simulink library "fcnLib4joint_sim"  (R2018b)
settings: Solver=VariableStepAuto  StartTime=0.0  StopTime=10.0  RelTol=1e-3
values from neighbouring files (symbols this model uses):
  alpha = 1.0    (= 1)    [init.m]
  D_el = 0    [init.m]
  F_c = 35    [init.m]
  F_s = 40    [init.m]
  J_joint = 4.155    [init.m]
  J_load = 1.2252    [init.m]
  K0_colli = 100    [init.m]
  K_el = 6900    [init.m]
  L_fricObs = 50    [init.m]
  sigma0 = 2000    [init.m]
  sigma1 = 200    [init.m]
  sigma2 = D_visc    (= 20)    [init.m]
  vs = 0.1    [init.m]
undefined symbols (not defined in the file or in its folder): threshold_colli, X, Y, Z
libraries: fl_lib x22, nesl_utility x16, sm_lib x6, simulink x4, sdl_lib x2, dsparch4 x1
settings Model: Creator=qiming  LastModifiedBy=qiming

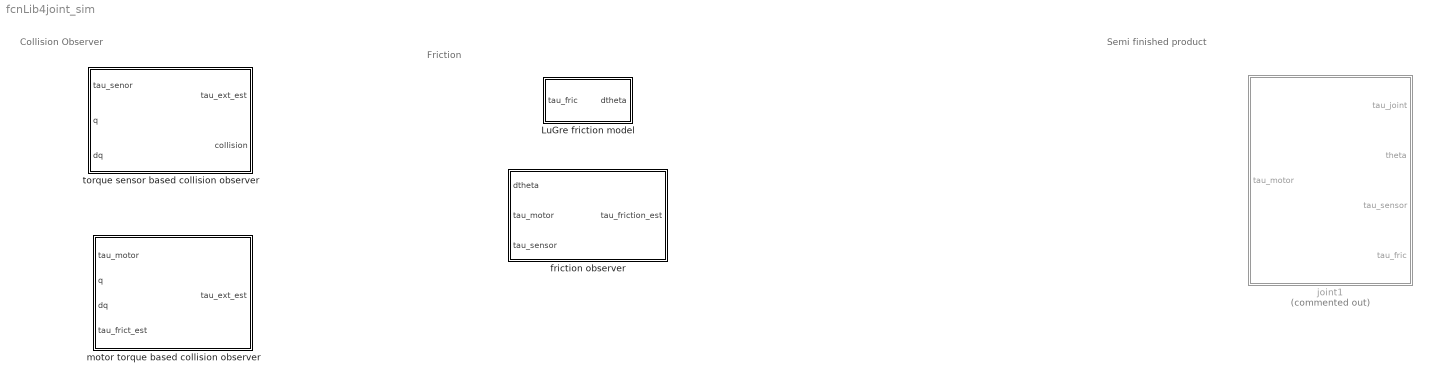
== system fcnLib4joint_sim ==
  note: Semi finished product
  note: Friction
  note: Collision Observer
  " torque sensor based collision observer " : Subsystem
  LuGre friction model : Subsystem
  friction observer : Subsystem
  joint1 : Subsystem  Commented=on
  motor torque based collision observer : Subsystem

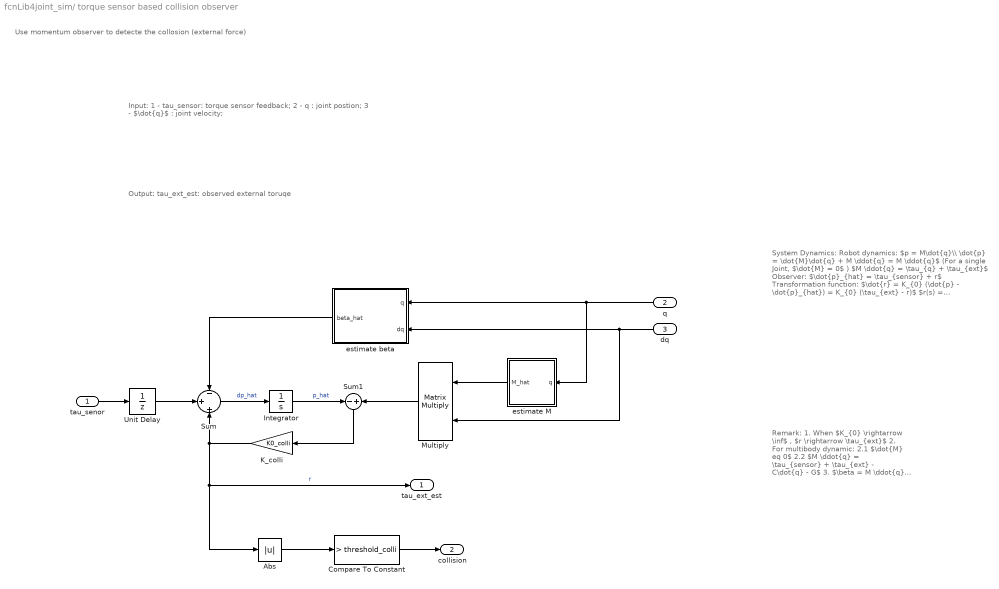
== system fcnLib4joint_sim/ torque sensor based collision observer  ==
  note: Input:
      | 1 - tau_sensor: torque sensor feedback;
      | 2 - q : joint postion;
      | 3 - $\dot{q}$ : joint velocity;
  note: Use momentum observer to detecte the collosion (external force)
  note: Output:
      | tau_ext_est: observed external toruqe
  note: System Dynamics:
      | Robot dynamics:
      | $p = M\dot{q}\\ \dot{p} = \dot{M}\dot{q} + M \ddot{q} = M \ddot{q}$ (For a single Joint, $\dot{M} = 0$ )
      | $M \ddot{q} = \tau_{q} + \tau_{ext}$
      | Observer:
      | $\dot{p}_{hat} = \tau_{sensor} + r$
      | Transformation function:
      | $\dot{r} = K_{0} (\dot{p} - \dot{p}_{hat}) = K_{0} (\tau_{ext} - r)$
      | $r(s) = \frac{1}{1+\frac{1}{K_{0}}s} \tau_{ext}(s)$
  note: Remark:
      | 1. When $K_{0} \rightarrow \inf$ , $r \rightarrow \tau_{ext}$
      | 2. For multibody dynamic:
      | 2.1 $\dot{M} \neq 0$
      | 2.2 $M \ddot{q} = \tau_{sensor} + \tau_{ext} - C\dot{q} - G$
      | 3. $\beta = M \ddot{q} = C\dot{q} + G$
  tau_senor : Inport
  q : Inport  Port=2
  dq : Inport  Port=3
  Abs : Abs
  Compare To Constant : simulink/Logic and Bit Operations/Compare To Constant  relop=>  const=threshold_colli  OutDataTypeStr=boolean
  Integrator : Integrator
  K_colli : Gain  Gain=K0_colli
  Multiply : Product  Multiplication=Matrix(*)
  Sum : Sum  Inputs=-|+|+
  Sum1 : Sum  Inputs=-+
  Unit Delay : UnitDelay  SampleTime=-1
  estimate M : Subsystem
  "estimate beta " : Subsystem
  tau_ext_est : Outport
  collision : Outport  Port=2
  wires:
  tau_senor/1 -> Unit Delay/1
  q/1 -> estimate M/1(q), "estimate beta "/1(q)
  "estimate beta "/1(beta_hat) -> Sum/1
  Sum/1 -> Integrator/1  "dp_hat"
  Integrator/1 -> Sum1/1  "p_hat"
  estimate M/1(M_hat) -> Multiply/1
  dq/1 -> Multiply/2, "estimate beta "/2(dq)
  K_colli/1 -> Abs/1, tau_ext_est/1, Sum/3  "r"
  Sum1/1 -> K_colli/1
  Compare To Constant/1 -> collision/1
  Abs/1 -> Compare To Constant/1
  Multiply/1 -> Sum1/2
  Unit Delay/1 -> Sum/2

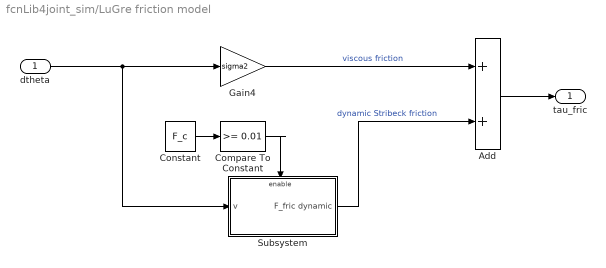
== system fcnLib4joint_sim/LuGre friction model ==
  dtheta : Inport
  Add : Sum
  Compare To Constant : simulink/Logic and Bit Operations/Compare To Constant  relop=>=  const=0.01  OutDataTypeStr=boolean
  Constant : Constant  Value=F_c
  Gain4 : Gain  Gain=sigma2
  Subsystem : Subsystem
  tau_fric : Outport
  wires:
  dtheta/1 -> Subsystem/1(v), Gain4/1
  Gain4/1 -> Add/1  "viscous friction"
  Add/1 -> tau_fric/1
  Constant/1 -> Compare To Constant/1
  Compare To Constant/1 -> Subsystem/Enable
  Subsystem/1(F_fric dynamic) -> Add/2  "dynamic Stribeck friction"

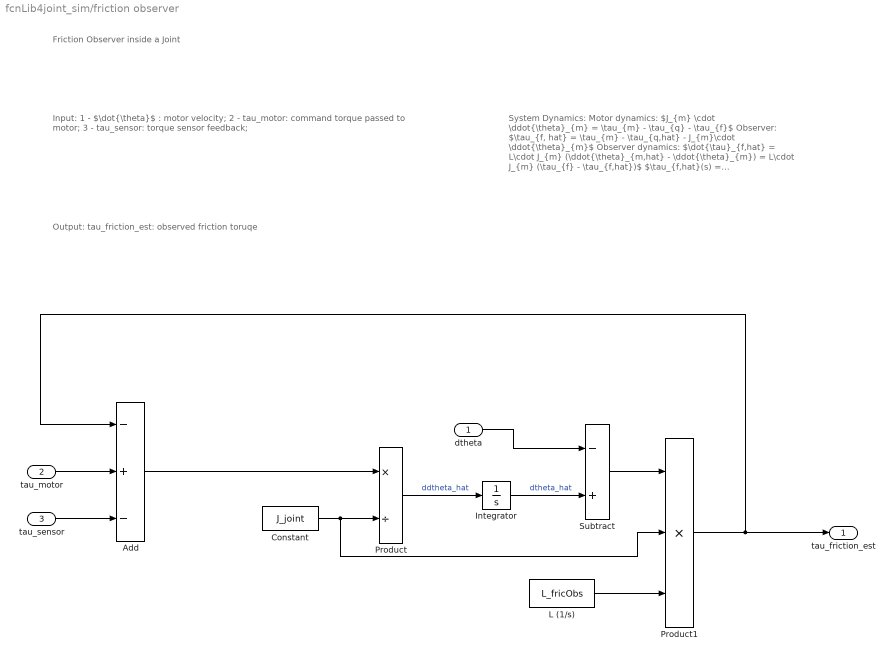
== system fcnLib4joint_sim/friction observer ==
  note: Friction Observer inside a Joint
  note: Output:
      | tau_friction_est: observed friction toruqe
  note: Input:
      | 1 - $\dot{\theta}$ : motor velocity;
      | 2 - tau_motor: command torque passed to motor;
      | 3 - tau_sensor: torque sensor feedback;
  note: System Dynamics:
      | Motor dynamics:
      | $J_{m} \cdot \ddot{\theta}_{m} = \tau_{m} - \tau_{q} - \tau_{f}$
      | Observer:
      | $\tau_{f, hat} = \tau_{m} - \tau_{q,hat} - J_{m}\cdot \ddot{\theta}_{m}$
      | Observer dynamics:
      | $\dot{\tau}_{f,hat} = L\cdot J_{m} (\ddot{\theta}_{m,hat} - \ddot{\theta}_{m}) = L\cdot J_{m} (\tau_{f} - \tau_{f,hat})$
      | $\tau_{f,hat}(s) = \frac{1}{1+\frac{1}{L\cdot J_{m}}s} \tau_{f}(s)$
  dtheta : Inport
  tau_motor : Inport  Port=2
  tau_sensor : Inport  Port=3
  Add : Sum  Inputs=-+-
  Constant : Constant  Value=J_joint
  Integrator : Integrator
  L (1/s) : Constant  Value=L_fricObs
  Product : Product  Inputs=*/
  Product1 : Product  Inputs=3
  Subtract : Sum  Inputs=-+
  tau_friction_est : Outport
  wires:
  Product/1 -> Integrator/1  "ddtheta_hat"
  Integrator/1 -> Subtract/2  "dtheta_hat"
  Constant/1 -> Product1/2, Product/2
  Subtract/1 -> Product1/1
  L (1/s)/1 -> Product1/3
  Add/1 -> Product/1
  Product1/1 -> tau_friction_est/1, Add/1
  dtheta/1 -> Subtract/1
  tau_motor/1 -> Add/2
  tau_sensor/1 -> Add/3

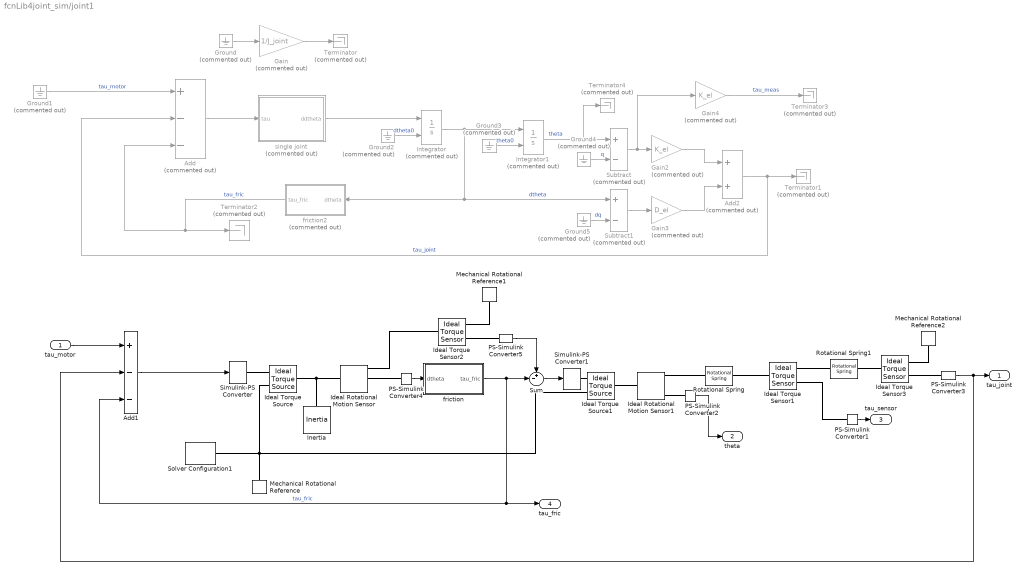
== system fcnLib4joint_sim/joint1 ==
  tau_motor : Inport
  Add : Sum  Commented=on  Inputs=+--
  Add1 : Sum  Inputs=+--
  Add2 : Sum  Commented=on
  Gain : Gain  Commented=on  Gain=1/J_joint
  Gain2 : Gain  Commented=on  Gain=K_el
  Gain3 : Gain  Commented=on  Gain=D_el
  Gain4 : Gain  Commented=on  Gain=K_el
  Ground{,1..5} (6 alike) : Ground  Commented=on
  Ideal Rotational Motion Sensor : fl_lib/Mechanical/Mechanical Sensors/Ideal Rotational Motion Sensor  offset=0 rad
  Ideal Rotational Motion Sensor1 : fl_lib/Mechanical/Mechanical Sensors/Ideal Rotational Motion Sensor  offset=0 rad
  Ideal Torque Sensor1 : fl_lib/Mechanical/Mechanical Sensors/Ideal Torque Sensor
  Ideal Torque Sensor2 : fl_lib/Mechanical/Mechanical Sensors/Ideal Torque Sensor
  Ideal Torque Sensor3 : fl_lib/Mechanical/Mechanical Sensors/Ideal Torque Sensor
  Ideal Torque Source : fl_lib/Mechanical/Mechanical Sources/Ideal Torque Source
  Ideal Torque Source1 : fl_lib/Mechanical/Mechanical Sources/Ideal Torque Source
  Inertia : fl_lib/Mechanical/Rotational Elements/Inertia  inertia=4.155 kg*m^2  w_specify=off  w_priority=High  w=0 rad/s  w_nominal_specify=off  w_nominal_unit=rad/s  w_nominal_value=1  t_specify=off  t_priority=None  t=0 N*m  t_nominal_specify=off  t_nominal_unit=N*m  t_nominal_value=1
  Integrator : Integrator  Commented=on  InitialConditionSource=external
  Integrator1 : Integrator  Commented=on  InitialConditionSource=external
  Mechanical Rotational Reference : fl_lib/Mechanical/Rotational Elements/Mechanical Rotational Reference
  Mechanical Rotational Reference1 : fl_lib/Mechanical/Rotational Elements/Mechanical Rotational Reference
  Mechanical Rotational Reference2 : fl_lib/Mechanical/Rotational Elements/Mechanical Rotational Reference
  PS-Simulink Converter{1..5} (5 alike) : nesl_utility/PS-Simulink Converter  PhysicalDomain=network_engine_domain  SubClassName=ps_output  LeftPortType=input  RightPortType=output  PseudoPeriodic=off  Frequencies=[]  Unit=1  AffineConversion=off
  Rotational Spring : fl_lib/Mechanical/Rotational Elements/Rotational Spring  spr_rate=6900 N*m/rad  w_specify=off  w_priority=None  w=0 rad/s  w_nominal_specify=off  w_nominal_unit=rad/s  w_nominal_value=1  t_specify=off  t_priority=None  t=0 N*m  t_nominal_specify=off  t_nominal_unit=N*m  t_nominal_value=1  phi_specify=off  phi_priority=High  phi=0 rad  phi_nominal_specify=off  phi_nominal_unit=rad  phi_nominal_value=1
      settings: SourceProductName=Simscape
  Rotational Spring1 : fl_lib/Mechanical/Rotational Elements/Rotational Spring  spr_rate=6900 N*m/rad  w_specify=off  w_priority=None  w=0 rad/s  w_nominal_specify=off  w_nominal_unit=rad/s  w_nominal_value=1  t_specify=off  t_priority=None  t=0 N*m  t_nominal_specify=off  t_nominal_unit=N*m  t_nominal_value=1  phi_specify=off  phi_priority=High  phi=0 rad  phi_nominal_specify=off  phi_nominal_unit=rad  phi_nominal_value=1
      settings: SourceProductName=Simscape
  Simulink-PS Converter : nesl_utility/Simulink-PS Converter  PhysicalDomain=network_engine_domain  SubClassName=ps_input  LeftPortType=input  RightPortType=output  PseudoPeriodic=off  Frequencies=[]  NoiseDistribution=none  NoiseParameters=[]  Unit=1  AffineConversion=off  FilteringAndDerivatives=provide  SimscapeFilterOrder=1  InputFilterTimeConstant=0.001  UdotUserProvided=0
  Simulink-PS Converter1 : nesl_utility/Simulink-PS Converter  PhysicalDomain=network_engine_domain  SubClassName=ps_input  LeftPortType=input  RightPortType=output  PseudoPeriodic=off  Frequencies=[]  NoiseDistribution=none  NoiseParameters=[]  Unit=1  AffineConversion=off  FilteringAndDerivatives=provide  SimscapeFilterOrder=1  InputFilterTimeConstant=0.001  UdotUserProvided=0
  Solver Configuration1 : nesl_utility/Solver Configuration  PhysicalDomain=network_engine_domain  SubClassName=solver  LeftPortType=input  RightPortType=generic  Tones=[]  Harmonics=[]  SimulateNoise=off  Profile=off  UseLocalSampling=off  EnableSwitchedLinearOptims=on  FrequencyDomain=off  UseCCode=off  RelTol=0.001  AbsTol=1e-06  MinStep=1e-09  ToWorkspace=off  RevertToSquareIcSolve=off  NumHomotopyIterations=100  PhasorMode=off  PhasorModeNumHarmonics=1  DoDC=off  ResidualTolerance=1e-09  UseLocalSolver=off  LocalSolverChoice=NE_BACKWARD_EULER_ADVANCER  LocalSolverSampleTime=0.001  DoFixedCost=off  MaxNonlinIter=3  MaxModeIter=2  LinearAlgebra=auto  EquationFormulation=NE_TIME_EF  DelaysMemoryBudget=1024  AutomaticFiltering=on  FilteringTimeConstant=0.001  PartitionStorageMethod=AS_NEEDED  PartitionMemoryBudget=1024
  Subtract : Sum  Commented=on  Inputs=+-
  Subtract1 : Sum  Commented=on  Inputs=+-
  Sum : Sum  Inputs=+-|
  Terminator{,1..4} (5 alike) : Terminator  Commented=on
  friction : Subsystem
  friction2 : Subsystem  Commented=on
  single joint : Subsystem  Commented=on
  tau_joint : Outport
  theta : Outport  Port=2
  tau_sensor : Outport  Port=3
  tau_fric : Outport  Port=4
  wires:
  Ground4/1 -> Subtract/2  "q"
  Gain4/1 -> Terminator3/1  "tau_meas"
  Gain3/1 -> Add2/2
  Gain2/1 -> Add2/1
  Add2/1 -> Add/2, Terminator1/1  "tau_joint"
  Ground3/1 -> Integrator1/2  "theta0"
  Integrator/1 -> Integrator1/1, Subtract1/1, friction2/1(dtheta)  "dtheta"
  Subtract/1 -> Gain4/1, Gain2/1
  Subtract1/1 -> Gain3/1
  Integrator1/1 -> Terminator4/1, Subtract/1  "theta"
  Ground2/1 -> Integrator/2  "dtheta0"
  friction2/1(tau_fric) -> Add/3, Terminator2/1  "tau_fric"
  Ground5/1 -> Subtract1/2  "dq"
  Ground/1 -> Gain/1
  Gain/1 -> Terminator/1
  PS-Simulink Converter3/1 -> tau_joint/1, Add1/2
  PS-Simulink Converter1/1 -> tau_sensor/1
  single joint/1(ddtheta) -> Integrator/1
  Ground1/1 -> Add/1  "tau_motor"
  Add/1 -> single joint/1(tau)
  PS-Simulink Converter4/1 -> friction/1(dtheta)
  friction/1(tau_fric) -> Sum/2, Add1/3, tau_fric/1  "tau_fric"
  PS-Simulink Converter5/1 -> Sum/1
  Sum/1 -> Simulink-PS Converter1/1
  PS-Simulink Converter2/1 -> theta/1
  tau_motor/1 -> Add1/1
  Add1/1 -> Simulink-PS Converter/1
  connections:
  Ideal Rotational Motion Sensor/RConn1 -- Ideal Torque Sensor2/LConn1
  Solver Configuration1/RConn1 -- Mechanical Rotational Reference/LConn1 -- Ideal Torque Source1/RConn2 -- Ideal Torque Source/RConn2
  PS-Simulink Converter3/LConn1 -- Ideal Torque Sensor3/RConn2
  Simulink-PS Converter/RConn1 -- Ideal Torque Source/RConn1
  Inertia/LConn1 -- Ideal Rotational Motion Sensor/LConn1 -- Ideal Torque Source/LConn1
  PS-Simulink Converter4/LConn1 -- Ideal Rotational Motion Sensor/RConn2
  Ideal Torque Sensor2/RConn1 -- Mechanical Rotational Reference1/LConn1
  PS-Simulink Converter5/LConn1 -- Ideal Torque Sensor2/RConn2
  Ideal Torque Source1/RConn1 -- Simulink-PS Converter1/RConn1
  Ideal Rotational Motion Sensor1/LConn1 -- Ideal Torque Source1/LConn1
  PS-Simulink Converter2/LConn1 -- Ideal Rotational Motion Sensor1/RConn3
  Rotational Spring/LConn1 -- Ideal Rotational Motion Sensor1/RConn1
  Ideal Torque Sensor1/LConn1 -- Rotational Spring/RConn1
  Rotational Spring1/LConn1 -- Ideal Torque Sensor1/RConn1
  Ideal Torque Sensor3/LConn1 -- Rotational Spring1/RConn1
  PS-Simulink Converter1/LConn1 -- Ideal Torque Sensor1/RConn2
  Mechanical Rotational Reference2/LConn1 -- Ideal Torque Sensor3/RConn1

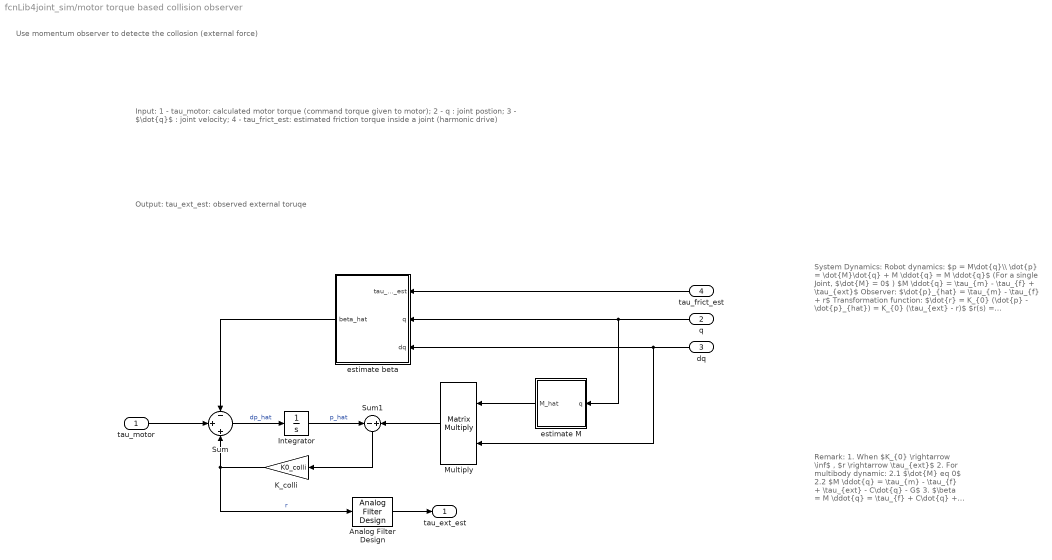
== system fcnLib4joint_sim/motor torque based collision observer ==
  note: Input:
      | 1 - tau_motor: calculated motor torque (command torque given to motor);
      | 2 - q : joint postion;
      | 3 - $\dot{q}$ : joint velocity;
      | 4 - tau_frict_est: estimated friction torque inside a joint (harmonic drive)
  note: Use momentum observer to detecte the collosion (external force)
  note: Output:
      | tau_ext_est: observed external toruqe
  note: System Dynamics:
      | Robot dynamics:
      | $p = M\dot{q}\\ \dot{p} = \dot{M}\dot{q} + M \ddot{q} = M \ddot{q}$ (For a single Joint, $\dot{M} = 0$ )
      | $M \ddot{q} = \tau_{m} - \tau_{f} + \tau_{ext}$
      | Observer:
      | $\dot{p}_{hat} = \tau_{m} - \tau_{f} + r$
      | Transformation function:
      | $\dot{r} = K_{0} (\dot{p} - \dot{p}_{hat}) = K_{0} (\tau_{ext} - r)$
      | $r(s) = \frac{1}{1+\frac{1}{K_{0}}s} \tau_{ext}(s)$
  note: Remark:
      | 1. When $K_{0} \rightarrow \inf$ , $r \rightarrow \tau_{ext}$
      | 2. For multibody dynamic:
      | 2.1 $\dot{M} \neq 0$
      | 2.2 $M \ddot{q} = \tau_{m} - \tau_{f} + \tau_{ext} - C\dot{q} - G$
      | 3. $\beta = M \ddot{q} = \tau_{f} + C\dot{q} + G$
  tau_motor : Inport
  q : Inport  Port=2
  dq : Inport  Port=3
  tau_frict_est : Inport  Port=4
  Analog Filter Design : dsparch4/Analog Filter Design  method=Butterworth  filttype=Lowpass  N=2  Wlo=30  Whi=80  Rp=2  Rs=20
  Integrator : Integrator
  K_colli : Gain  Gain=K0_colli
  Multiply : Product  Multiplication=Matrix(*)
  Sum : Sum  Inputs=-|+|+
  Sum1 : Sum  Inputs=-+
  estimate M : Subsystem
  "estimate beta " : Subsystem
  tau_ext_est : Outport
  wires:
  tau_motor/1 -> Sum/2
  q/1 -> estimate M/1(q), "estimate beta "/2(q)
  "estimate beta "/1(beta_hat) -> Sum/1
  Sum/1 -> Integrator/1  "dp_hat"
  Integrator/1 -> Sum1/1  "p_hat"
  estimate M/1(M_hat) -> Multiply/1
  dq/1 -> Multiply/2, "estimate beta "/3(dq)
  Multiply/1 -> Sum1/2
  Analog Filter Design/1 -> tau_ext_est/1
  K_colli/1 -> Analog Filter Design/1, Sum/3  "r"
  Sum1/1 -> K_colli/1
  tau_frict_est/1 -> "estimate beta "/1(tau_fric_est)

== system fcnLib4joint_sim/ torque sensor based collision observer /estimate M ==
  q : Inport
  Constant : Constant  Value=J_load
  Terminator : Terminator
  M_hat : Outport
  wires:
  Constant/1 -> M_hat/1
  q/1 -> Terminator/1

== system fcnLib4joint_sim/ torque sensor based collision observer /estimate beta  ==
  q : Inport
  dq : Inport  Port=2
  Ground : Ground
  Terminator : Terminator
  Terminator1 : Terminator
  beta_hat : Outport
  wires:
  dq/1 -> Terminator/1
  q/1 -> Terminator1/1
  Ground/1 -> beta_hat/1

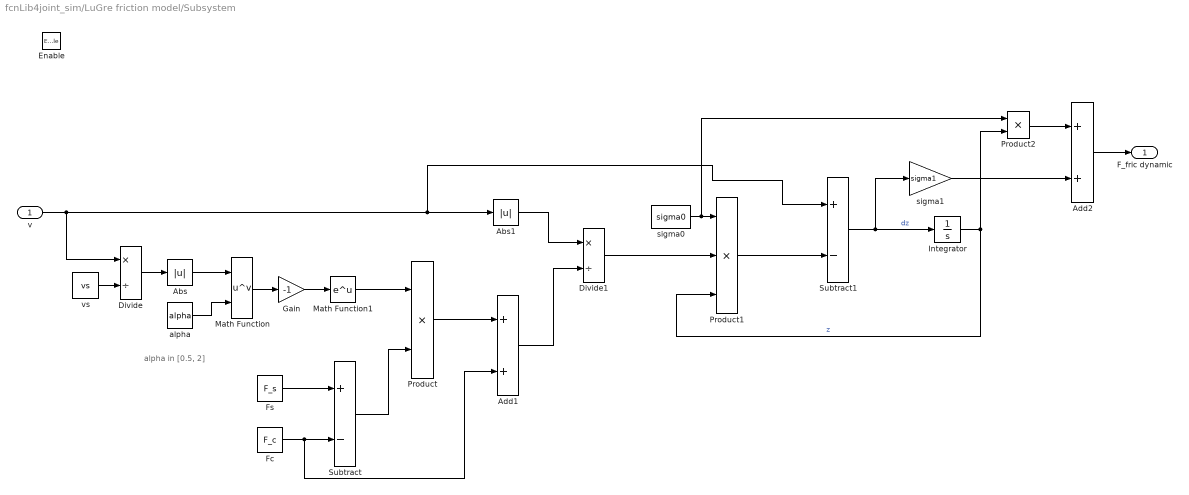
== system fcnLib4joint_sim/LuGre friction model/Subsystem ==
  note: alpha in [0.5, 2]
  v : Inport
  Enable : EnablePort  StatesWhenEnabling=reset
  Abs : Abs
  Abs1 : Abs
  Add1 : Sum
  Add2 : Sum
  Divide : Product  Inputs=*/
  Divide1 : Product  Inputs=*/
  Fc : Constant  Value=F_c
  Fs : Constant  Value=F_s
  Gain : Gain  Gain=-1
  Integrator : Integrator
  Math Function : Math  Operator=pow  SaturateOnIntegerOverflow=on
  Math Function1 : Math  SaturateOnIntegerOverflow=on
  Product : Product
  Product1 : Product  Inputs=3
  Product2 : Product
  Subtract : Sum  Inputs=+-
  Subtract1 : Sum  Inputs=+-
  alpha : Constant  Value=alpha
  sigma0 : Constant  Value=sigma0
  sigma1 : Gain  Gain=sigma1
  vs : Constant  Value=vs
  F_fric dynamic : Outport  OutputWhenDisabled=reset  InitialOutput=0
  wires:
  Product1/1 -> Subtract1/2
  Divide1/1 -> Product1/2
  Abs/1 -> Math Function/1
  sigma1/1 -> Add2/2
  sigma0/1 -> Product2/1, Product1/1
  v/1 -> Subtract1/1, Abs1/1, Divide/1
  Product2/1 -> Add2/1
  Product/1 -> Add1/1
  Subtract/1 -> Product/2
  Math Function1/1 -> Product/1
  Divide/1 -> Abs/1
  alpha/1 -> Math Function/2
  Integrator/1 -> Product2/2, Product1/3  "z"
  Gain/1 -> Math Function1/1
  Fc/1 -> Add1/2, Subtract/2
  vs/1 -> Divide/2
  Subtract1/1 -> sigma1/1, Integrator/1  "dz"
  Math Function/1 -> Gain/1
  Add1/1 -> Divide1/2
  Abs1/1 -> Divide1/1
  Fs/1 -> Subtract/1
  Add2/1 -> F_fric dynamic/1

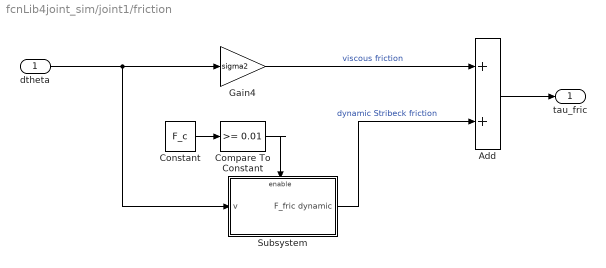
== system fcnLib4joint_sim/joint1/friction ==
  dtheta : Inport
  Add : Sum
  Compare To Constant : simulink/Logic and Bit Operations/Compare To Constant  relop=>=  const=0.01  OutDataTypeStr=boolean
  Constant : Constant  Value=F_c
  Gain4 : Gain  Gain=sigma2
  Subsystem : Subsystem
  tau_fric : Outport
  wires:
  dtheta/1 -> Subsystem/1(v), Gain4/1
  Gain4/1 -> Add/1  "viscous friction"
  Add/1 -> tau_fric/1
  Constant/1 -> Compare To Constant/1
  Compare To Constant/1 -> Subsystem/Enable
  Subsystem/1(F_fric dynamic) -> Add/2  "dynamic Stribeck friction"

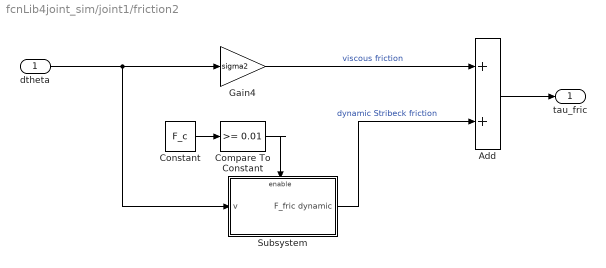
== system fcnLib4joint_sim/joint1/friction2 ==
  dtheta : Inport
  Add : Sum
  Compare To Constant : simulink/Logic and Bit Operations/Compare To Constant  relop=>=  const=0.01  OutDataTypeStr=boolean
  Constant : Constant  Value=F_c
  Gain4 : Gain  Gain=sigma2
  Subsystem : Subsystem
  tau_fric : Outport
  wires:
  dtheta/1 -> Subsystem/1(v), Gain4/1
  Gain4/1 -> Add/1  "viscous friction"
  Add/1 -> tau_fric/1
  Constant/1 -> Compare To Constant/1
  Compare To Constant/1 -> Subsystem/Enable
  Subsystem/1(F_fric dynamic) -> Add/2  "dynamic Stribeck friction"

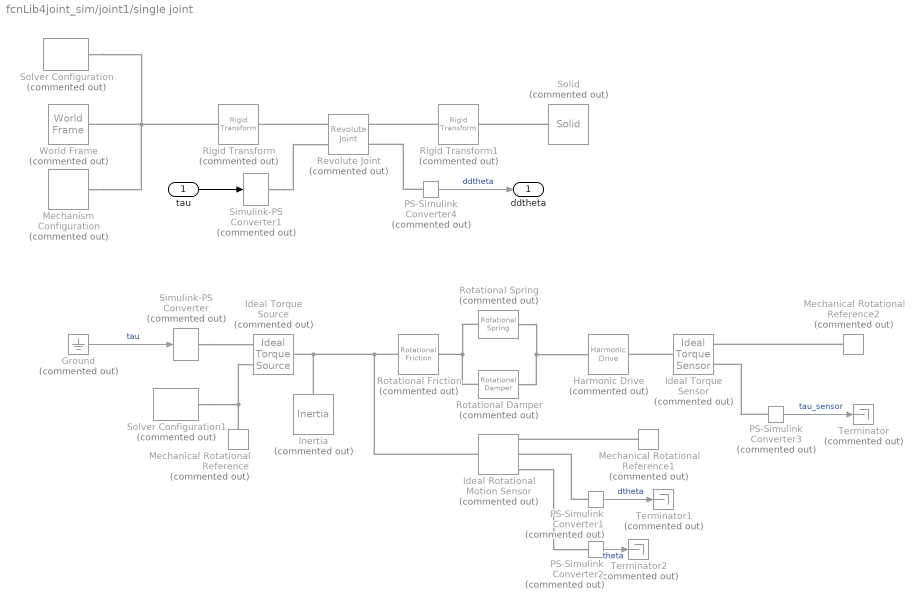
== system fcnLib4joint_sim/joint1/single joint ==
  tau : Inport
  Ground : Ground  Commented=on
  Harmonic Drive : sdl_lib/Gears/Harmonic Drive  Commented=on  n_ellipse=100  n_circle=102  friction_model=1  T_noload=0.1 N*m  T_nom=5 N*m  efficiency_nom=.95  efficiency=.95  mu_visc=[0, 0] N*m/(rad/s)  w_thr=0.01 rad/s  pwr_thr=0.001 W  temperature_TLU=[280, 300, 320] K  load_TLU=[1, 5, 10] N*m  efficiency_TLU=[.95, .9, .85]  efficiency_TLU2=[.85, .8, .75; .95, .9, .85; .85, .8, .7]  thermal_mass=50 J/K  T_init=300 K
      settings: SourceProductName=Simscape Driveline  SourceProductBaseCode=LD
  Ideal Rotational Motion Sensor : fl_lib/Mechanical/Mechanical Sensors/Ideal Rotational Motion Sensor  Commented=on  offset=0 rad
  Ideal Torque Sensor : fl_lib/Mechanical/Mechanical Sensors/Ideal Torque Sensor  Commented=on
  Ideal Torque Source : fl_lib/Mechanical/Mechanical Sources/Ideal Torque Source  Commented=on
  Inertia : fl_lib/Mechanical/Rotational Elements/Inertia  Commented=on  inertia=0.01 kg*m^2  w_specify=off  w_priority=High  w=0 rad/s  w_nominal_specify=off  w_nominal_unit=rad/s  w_nominal_value=1  t_specify=off  t_priority=None  t=0 N*m  t_nominal_specify=off  t_nominal_unit=N*m  t_nominal_value=1
  Mechanical Rotational Reference : fl_lib/Mechanical/Rotational Elements/Mechanical Rotational Reference  Commented=on
  Mechanical Rotational Reference1 : fl_lib/Mechanical/Rotational Elements/Mechanical Rotational Reference  Commented=on
  Mechanical Rotational Reference2 : fl_lib/Mechanical/Rotational Elements/Mechanical Rotational Reference  Commented=on
  Mechanism Configuration : sm_lib/Utilities/Mechanism Configuration  Commented=on  UniformGravity=Constant  GravityVector=[0 0 -9.80665]  GravityUnits=m/s^2  LinearizationDelta=0.001
  PS-Simulink Converter{1..4} (4 alike) : nesl_utility/PS-Simulink Converter  Commented=on  PhysicalDomain=network_engine_domain  SubClassName=ps_output  LeftPortType=input  RightPortType=output  PseudoPeriodic=off  Frequencies=[]  Unit=1  AffineConversion=off
  Revolute Joint : sm_lib/Joints/Revolute Joint  Commented=on  SenseConstraintForce=off  SenseConstraintForceX=off  SenseConstraintForceY=off  SenseConstraintForceZ=off  SenseConstraintTorque=off  SenseConstraintTorqueX=off  SenseConstraintTorqueY=off  SenseConstraintTorqueZ=off  SenseTotalForce=off  SenseTotalForceX=off  SenseTotalForceY=off  SenseTotalForceZ=off  SenseTotalTorque=off  SenseTotalTorqueX=off  SenseTotalTorqueY=off  SenseTotalTorqueZ=off  CompositeWrenchDir=FollowerOnBase  CompositeWrenchFrame=BaseFrame  EquilibriumPosition=0  EquilibriumPositionUnits=deg  SpringStiffness=0  SpringStiffnessUnits=N*m/deg  DampingCoefficient=0  DampingCoefficientUnits=N*m/(deg/s)  TorqueActuationMode=InputTorque  MotionActuationMode=ComputedMotion  SensePosition=off  SenseVelocity=off  SenseAcceleration=on  SenseTorqueForce=off  PositionTargetSpecify=off  PositionTargetPriority=High  PositionTargetValue=0  PositionTargetValueUnits=deg  VelocityTargetSpecify=off  VelocityTargetPriority=High  VelocityTargetValue=0  VelocityTargetValueUnits=deg/s
  Rigid Transform : sm_lib/Frames and Transforms/Rigid Transform  Commented=on  TranslationMethod=None  TranslationStandardOffset=150  TranslationLengthUnit=mm  TranslationStandardAxis=-X  TranslationCartesianOffset=[-150 0 0]  TranslationROffset=0  TranslationROffsetUnits=m  TranslationZOffset=0  TranslationZOffsetUnits=m  TranslationThetaOffset=0  TranslationThetaOffsetUnits=deg  RotationMethod=None  RotationAngleUnits=deg  RotationStandardAxis=+Z  RotationAngle=0.0  RotationArbitraryAxis=[0 0 1]  FollAlignAxisA=+X  BaseAlignAxisA=+Y  FollAlignAxisB=+Y  BaseAlignAxisB=+Z  RotationSequenceAxes=FollowerAxes  RotationSequence=XYX  RotationSequenceAngles=[0 0 0]  RotationSequenceAnglesUnits=deg  RotationMatrix=[1 0 0; 0 1 0; 0 0 1]
  Rigid Transform1 : sm_lib/Frames and Transforms/Rigid Transform  Commented=on  TranslationMethod=StandardAxis  TranslationStandardOffset=150  TranslationLengthUnit=mm  TranslationStandardAxis=+X  TranslationCartesianOffset=[0 0 0]  TranslationROffset=0  TranslationROffsetUnits=m  TranslationZOffset=0  TranslationZOffsetUnits=m  TranslationThetaOffset=0  TranslationThetaOffsetUnits=deg  RotationMethod=None  RotationAngleUnits=deg  RotationStandardAxis=+Z  RotationAngle=0.0  RotationArbitraryAxis=[0 0 1]  FollAlignAxisA=+X  BaseAlignAxisA=+Y  FollAlignAxisB=+Y  BaseAlignAxisB=+Z  RotationSequenceAxes=FollowerAxes  RotationSequence=XYX  RotationSequenceAngles=[0 0 0]  RotationSequenceAnglesUnits=deg  RotationMatrix=[1 0 0; 0 1 0; 0 0 1]
  Rotational Damper : sdl_lib/Couplings & Drives/Springs & Dampers/Rotational Damper  Commented=on  D=1e-3 N*m/(rad/s)  enable_faults=0  b_fault=100 N*m/(rad/s)  temporal_fault=0  fault_time=5 s  shock_fault=0  acceleration_limit=100 rad/s^2  shock_limit=1  report_fault=1
      settings: SourceProductName=Simscape Driveline  SourceProductBaseCode=LD
  Rotational Friction : fl_lib/Mechanical/Rotational Elements/Rotational Friction  Commented=on  brkwy_trq=25 N*m  brkwy_vel=0.1 rad/s  Col_trq=20 N*m  visc_coef=0.001 N*m/(rad/s)  w_specify=off  w_priority=None  w=0 rad/s  w_nominal_specify=off  w_nominal_unit=rad/s  w_nominal_value=1  t_specify=off  t_priority=None  t=0 N*m  t_nominal_specify=off  t_nominal_unit=N*m  t_nominal_value=1
      settings: SourceProductName=Simscape
  Rotational Spring : fl_lib/Mechanical/Rotational Elements/Rotational Spring  Commented=on  spr_rate=10 N*m/rad  w_specify=off  w_priority=None  w=0 rad/s  w_nominal_specify=off  w_nominal_unit=rad/s  w_nominal_value=1  t_specify=off  t_priority=None  t=0 N*m  t_nominal_specify=off  t_nominal_unit=N*m  t_nominal_value=1  phi_specify=off  phi_priority=High  phi=0 rad  phi_nominal_specify=off  phi_nominal_unit=rad  phi_nominal_value=1
      settings: SourceProductName=Simscape
  Simulink-PS Converter : nesl_utility/Simulink-PS Converter  Commented=on  PhysicalDomain=network_engine_domain  SubClassName=ps_input  LeftPortType=input  RightPortType=output  PseudoPeriodic=off  Frequencies=[]  NoiseDistribution=none  NoiseParameters=[]  Unit=1  AffineConversion=off  FilteringAndDerivatives=provide  SimscapeFilterOrder=1  InputFilterTimeConstant=0.001  UdotUserProvided=0
  Simulink-PS Converter1 : nesl_utility/Simulink-PS Converter  Commented=on  PhysicalDomain=network_engine_domain  SubClassName=ps_input  LeftPortType=input  RightPortType=output  PseudoPeriodic=off  Frequencies=[]  NoiseDistribution=none  NoiseParameters=[]  Unit=1  AffineConversion=off  FilteringAndDerivatives=provide  SimscapeFilterOrder=1  InputFilterTimeConstant=0.001  UdotUserProvided=0
  Solid : sm_lib/Body Elements/Solid  Commented=on  InertiaType=Custom  Mass=1  MassUnits=kg  CenterOfMass=[0 0 0]  CenterOfMassUnits=m  MomentsOfInertia=[1 1 4.155]  MomentsOfInertiaUnits=kg*m^2  ProductsOfInertia=[0 0 0]  ProductsOfInertiaUnits=kg*m^2  BasedOnType=Density  Density=2700  DensityUnits=kg/m^3  DoExposeReferenceFrame=on  SerializedFrames=<Frames/>  GraphicType=FromGeometry  MarkerShape=Sphere  MarkerSize=10  GraphicVisPropType=SimpleVisualProperties  GraphicDiffuseColor=[0.5 0.5 0.5]  GraphicSpecularColor=[0.5 0.5 0.5 1.0]  GraphicAmbientColor=[0.15 0.15 0.15 1.0]  GraphicEmissiveColor=[0.0 0.0 0.0 1.0]  GraphicShininess=75  GraphicOpacity=1.0  GeometryShape=Brick  RectangleSize=[1 1]  RectangleSizeUnits=m  BrickDimensions=[300 30 30]  BrickDimensionUnits=mm  CylinderRadius=1  CylinderRadiusUnits=m  CylinderLength=1  CylinderLengthUnits=m  SphereRadius=1  SphereRadiusUnits=m  EllipsoidRadii=[1 1 1]  EllipsoidRadiiUnits=m  ExtrusionCrossSection=[1 1; -1 1; -1 -1; 1 -1]  ExtrusionCrossSectionUnits=m  ExtrusionLength=1  ExtrusionLengthUnits=m  PolygonNumSides=3  PolygonOuterRadius=1  PolygonOuterRadiusUnits=m  ExtGeomFileType=STEP  ExtGeomFileUnits=m  RevolutionCrossSection=[1 1; 1 -1; 2 -1; 2 1]  RevolutionCrossSectionUnits=m  RevolutionExtent=Full  RevolutionAngle=180  RevolutionAngleUnits=deg
  Solver Configuration : nesl_utility/Solver Configuration  Commented=on  PhysicalDomain=network_engine_domain  SubClassName=solver  LeftPortType=input  RightPortType=generic  Tones=[]  Harmonics=[]  SimulateNoise=off  Profile=off  UseLocalSampling=off  EnableSwitchedLinearOptims=on  FrequencyDomain=off  UseCCode=off  RelTol=0.001  AbsTol=1e-06  MinStep=1e-09  ToWorkspace=off  RevertToSquareIcSolve=off  NumHomotopyIterations=100  PhasorMode=off  PhasorModeNumHarmonics=1  DoDC=off  ResidualTolerance=1e-09  UseLocalSolver=off  LocalSolverChoice=NE_BACKWARD_EULER_ADVANCER  LocalSolverSampleTime=0.001  DoFixedCost=off  MaxNonlinIter=3  MaxModeIter=2  LinearAlgebra=auto  EquationFormulation=NE_TIME_EF  DelaysMemoryBudget=1024  AutomaticFiltering=on  FilteringTimeConstant=0.001  PartitionStorageMethod=AS_NEEDED  PartitionMemoryBudget=1024
  Solver Configuration1 : nesl_utility/Solver Configuration  Commented=on  PhysicalDomain=network_engine_domain  SubClassName=solver  LeftPortType=input  RightPortType=generic  Tones=[]  Harmonics=[]  SimulateNoise=off  Profile=off  UseLocalSampling=off  EnableSwitchedLinearOptims=on  FrequencyDomain=off  UseCCode=off  RelTol=0.001  AbsTol=1e-06  MinStep=1e-09  ToWorkspace=off  RevertToSquareIcSolve=off  NumHomotopyIterations=100  PhasorMode=off  PhasorModeNumHarmonics=1  DoDC=off  ResidualTolerance=1e-09  UseLocalSolver=off  LocalSolverChoice=NE_BACKWARD_EULER_ADVANCER  LocalSolverSampleTime=0.001  DoFixedCost=off  MaxNonlinIter=3  MaxModeIter=2  LinearAlgebra=auto  EquationFormulation=NE_TIME_EF  DelaysMemoryBudget=1024  AutomaticFiltering=on  FilteringTimeConstant=0.001  PartitionStorageMethod=AS_NEEDED  PartitionMemoryBudget=1024
  Terminator : Terminator  Commented=on
  Terminator1 : Terminator  Commented=on
  Terminator2 : Terminator  Commented=on
  World Frame : sm_lib/Frames and Transforms/World Frame  Commented=on
  ddtheta : Outport
  wires:
  PS-Simulink Converter2/1 -> Terminator2/1  "theta"
  PS-Simulink Converter1/1 -> Terminator1/1  "dtheta"
  PS-Simulink Converter3/1 -> Terminator/1  "tau_sensor"
  tau/1 -> Simulink-PS Converter1/1
  Ground/1 -> Simulink-PS Converter/1  "tau"
  PS-Simulink Converter4/1 -> ddtheta/1  "ddtheta"
  connections:
  PS-Simulink Converter4/LConn1 -- Revolute Joint/RConn2
  Solid/RConn1 -- Rigid Transform1/RConn1
  Revolute Joint/LConn1 -- Rigid Transform/RConn1
  Rigid Transform1/LConn1 -- Revolute Joint/RConn1
  Rigid Transform/LConn1 -- Solver Configuration/RConn1 -- Mechanism Configuration/RConn1 -- World Frame/RConn1
  Simulink-PS Converter1/RConn1 -- Revolute Joint/LConn2
  Simulink-PS Converter/RConn1 -- Ideal Torque Source/RConn1
  Mechanical Rotational Reference/LConn1 -- Solver Configuration1/RConn1 -- Ideal Torque Source/RConn2
  Rotational Friction/LConn1 -- Ideal Rotational Motion Sensor/LConn1 -- Inertia/LConn1 -- Ideal Torque Source/LConn1
  Rotational Spring/LConn1 -- Rotational Damper/LConn1 -- Rotational Friction/RConn1
  Rotational Spring/RConn1 -- Rotational Damper/RConn1 -- Harmonic Drive/LConn1
  Ideal Torque Sensor/LConn1 -- Harmonic Drive/RConn1
  PS-Simulink Converter1/LConn1 -- Ideal Rotational Motion Sensor/RConn2
  Ideal Rotational Motion Sensor/RConn3 -- PS-Simulink Converter2/LConn1
  Mechanical Rotational Reference1/LConn1 -- Ideal Rotational Motion Sensor/RConn1
  Mechanical Rotational Reference2/LConn1 -- Ideal Torque Sensor/RConn1
  PS-Simulink Converter3/LConn1 -- Ideal Torque Sensor/RConn2

== system fcnLib4joint_sim/motor torque based collision observer/estimate M ==
  q : Inport
  Add : Sum
  Constant : Constant  Value=J_load
  Constant1 : Constant  Value=J_joint
  Terminator : Terminator
  M_hat : Outport
  wires:
  Add/1 -> M_hat/1
  q/1 -> Terminator/1
  Constant/1 -> Add/1
  Constant1/1 -> Add/2

== system fcnLib4joint_sim/motor torque based collision observer/estimate beta  ==
  tau_fric_est : Inport
  q : Inport  Port=2
  dq : Inport  Port=3
  Terminator : Terminator
  Terminator1 : Terminator
  beta_hat : Outport
  wires:
  dq/1 -> Terminator/1
  q/1 -> Terminator1/1
  tau_fric_est/1 -> beta_hat/1

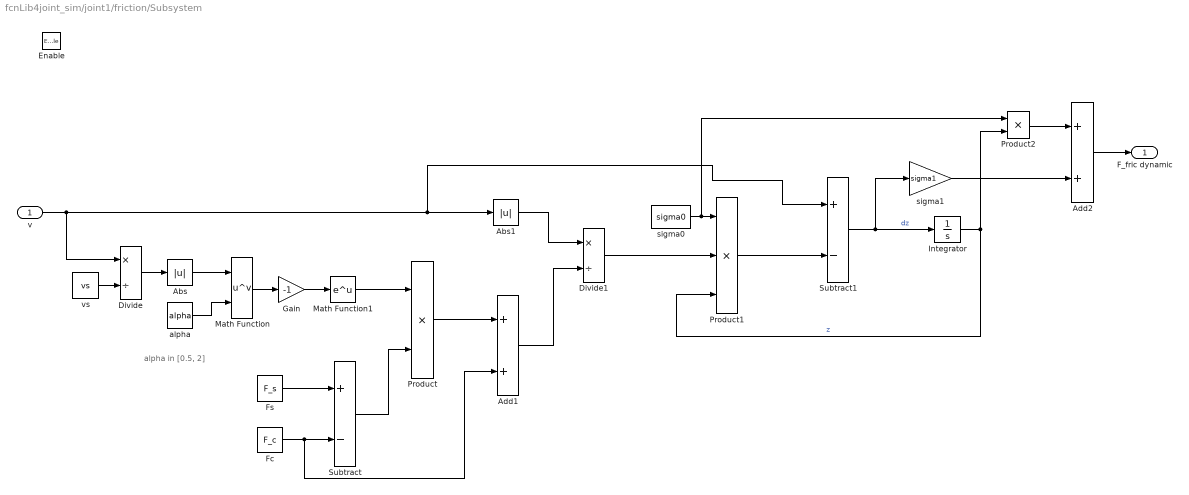
== system fcnLib4joint_sim/joint1/friction/Subsystem ==
  note: alpha in [0.5, 2]
  v : Inport
  Enable : EnablePort  StatesWhenEnabling=reset
  Abs : Abs
  Abs1 : Abs
  Add1 : Sum
  Add2 : Sum
  Divide : Product  Inputs=*/
  Divide1 : Product  Inputs=*/
  Fc : Constant  Value=F_c
  Fs : Constant  Value=F_s
  Gain : Gain  Gain=-1
  Integrator : Integrator
  Math Function : Math  Operator=pow  SaturateOnIntegerOverflow=on
  Math Function1 : Math  SaturateOnIntegerOverflow=on
  Product : Product
  Product1 : Product  Inputs=3
  Product2 : Product
  Subtract : Sum  Inputs=+-
  Subtract1 : Sum  Inputs=+-
  alpha : Constant  Value=alpha
  sigma0 : Constant  Value=sigma0
  sigma1 : Gain  Gain=sigma1
  vs : Constant  Value=vs
  F_fric dynamic : Outport  OutputWhenDisabled=reset  InitialOutput=0
  wires:
  Product1/1 -> Subtract1/2
  Divide1/1 -> Product1/2
  Abs/1 -> Math Function/1
  sigma1/1 -> Add2/2
  sigma0/1 -> Product2/1, Product1/1
  v/1 -> Subtract1/1, Abs1/1, Divide/1
  Product2/1 -> Add2/1
  Product/1 -> Add1/1
  Subtract/1 -> Product/2
  Math Function1/1 -> Product/1
  Divide/1 -> Abs/1
  alpha/1 -> Math Function/2
  Integrator/1 -> Product2/2, Product1/3  "z"
  Gain/1 -> Math Function1/1
  Fc/1 -> Add1/2, Subtract/2
  vs/1 -> Divide/2
  Subtract1/1 -> sigma1/1, Integrator/1  "dz"
  Math Function/1 -> Gain/1
  Add1/1 -> Divide1/2
  Abs1/1 -> Divide1/1
  Fs/1 -> Subtract/1
  Add2/1 -> F_fric dynamic/1

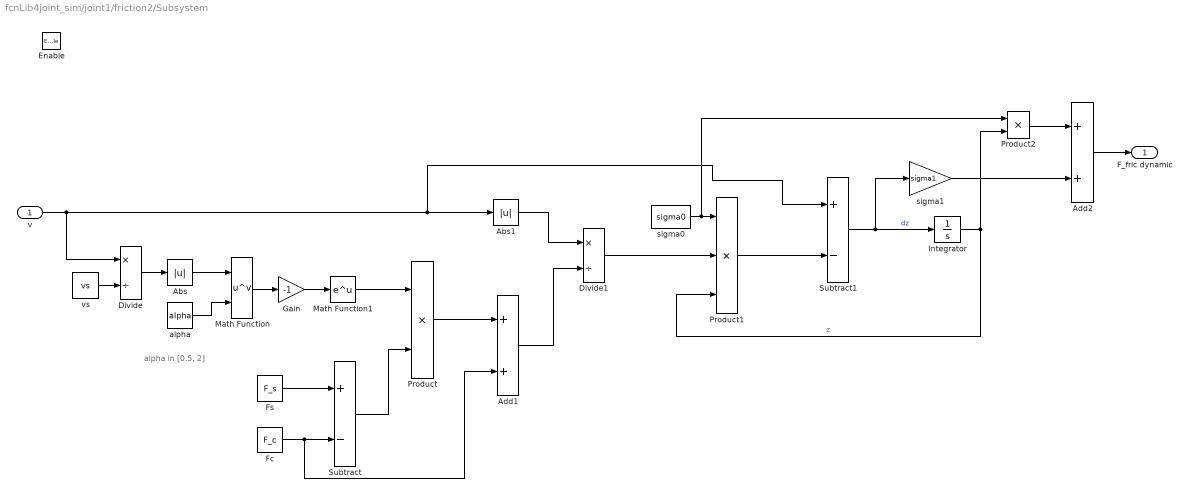
== system fcnLib4joint_sim/joint1/friction2/Subsystem ==
  note: alpha in [0.5, 2]
  v : Inport
  Enable : EnablePort  StatesWhenEnabling=reset
  Abs : Abs
  Abs1 : Abs
  Add1 : Sum
  Add2 : Sum
  Divide : Product  Inputs=*/
  Divide1 : Product  Inputs=*/
  Fc : Constant  Value=F_c
  Fs : Constant  Value=F_s
  Gain : Gain  Gain=-1
  Integrator : Integrator
  Math Function : Math  Operator=pow  SaturateOnIntegerOverflow=on
  Math Function1 : Math  SaturateOnIntegerOverflow=on
  Product : Product
  Product1 : Product  Inputs=3
  Product2 : Product
  Subtract : Sum  Inputs=+-
  Subtract1 : Sum  Inputs=+-
  alpha : Constant  Value=alpha
  sigma0 : Constant  Value=sigma0
  sigma1 : Gain  Gain=sigma1
  vs : Constant  Value=vs
  F_fric dynamic : Outport  OutputWhenDisabled=reset  InitialOutput=0
  wires:
  Product1/1 -> Subtract1/2
  Divide1/1 -> Product1/2
  Abs/1 -> Math Function/1
  sigma1/1 -> Add2/2
  sigma0/1 -> Product2/1, Product1/1
  v/1 -> Subtract1/1, Abs1/1, Divide/1
  Product2/1 -> Add2/1
  Product/1 -> Add1/1
  Subtract/1 -> Product/2
  Math Function1/1 -> Product/1
  Divide/1 -> Abs/1
  alpha/1 -> Math Function/2
  Integrator/1 -> Product2/2, Product1/3  "z"
  Gain/1 -> Math Function1/1
  Fc/1 -> Add1/2, Subtract/2
  vs/1 -> Divide/2
  Subtract1/1 -> sigma1/1, Integrator/1  "dz"
  Math Function/1 -> Gain/1
  Add1/1 -> Divide1/2
  Abs1/1 -> Divide1/1
  Fs/1 -> Subtract/1
  Add2/1 -> F_fric dynamic/1
